simulink subsystem "Independent_Suspension_Double_Wishbone"  (R2024b)
settings: Solver=VariableStepAuto  StartTime=0.0  StopTime=10.0  RelTol=1e-3
model mask{ActiveDampEn=off, NumAxl=2, NumWhlsByAxl=[2 2], StrgEnByAxl=[1 0], AntiSwayEnByAxl=[0 0], WhlNumVec=[1  2  1  2], AxleNumVec=[1  1  2  2], SuspTypesByAxle=[1  1], SuspImage=suspdw.png, IdealSuspEn=on, IdealSuspAxles=[1  2], Kz=64370, F0z=9810, Cz=10000, Hmax=0.5, f_act_susp_cz=[10000 10000;10000 10000], f_act_susp_duty_bpt=[0 1], f_act_susp_zdot_bpt=[-1 1], Toe=0.0349, RollStrgSlp=-0.2269, ToeStrgSlp=0.01, Caster=0.0698, CasterHslp=-0.2269, CasterStrgSlp=0.01, Camber=0.0698, CamberHslp=-0.2269, CamberStrgSlp=0.01, StrgHgtSlp=0.1432, MappedSuspEn=off, MappedSuspAxles=[1  2], f_susp_axl_bp=[1 2], f_susp_dz_bp=[-0.15 -0.14 -0.13 -0.12 -0.11 -0.10 -0.09 -0.08 -0.07 -0.06 -0.05 -0.04 -0.03 -0.02 -0.01 0.00 0.01 0.02 0.03 0.04 0.05 0.06 0.07 0.08 0.09 0.10 0.11 0.12 0.13 0.14 0.15], f_susp_dzdot_bp=[-0.15 -0.14 -0.13 -0.12 -0.11 -0.10 -0.09 -0.08 -0.07 -0.06 -0.05 -0.04 -0.03 -0.02 -0.01 0.00 0.01 0.02 0.03 0.04 0.05 0.06 0.07 0.08 0.09 0.10 0.11 0.12 0.13 0.14 0.15], f_susp_fmz=zeros(31,31,61,2,4), f_susp_geom=zeros(31,61,2,3), f_susp_strgdelta_bp=[-30,-29,-28,-27,-26,-25,-24,-23,-22,-21,-20,-19,-18,-17,-16,-15,-14,-13,-12,-11,-10,-9,-8,-7,-6,-5,-4,-3,-2,-1,0,1,2,3,4,5,6,7,8,9,10,11,12,13,14,15,16,17,18,19,20,21,22,23,24,25,26,27,28,29,30], AntiSwayR=0.2, AntiSwayNtrlAng=0.5236, AntiSwayTrsK=5.7296e+03}
  mask prompts: ActiveDampEn "vdynblks:vehdynDoubleWishboneSuspension:blkDlg_ActiveDampEn"; NumAxl "vdynblks:vehdynDoubleWishboneSuspension:blkPrm_NumAxl"; NumWhlsByAxl "vdynblks:vehdynDoubleWishboneSuspension:blkPrm_NumWhlsByAxl"; StrgEnByAxl "vdynblks:vehdynDoubleWishboneSuspension:blkPrm_StrgEnByAxl"; AntiSwayEnByAxl "vdynblks:vehdynDoubleWishboneSuspension:blkPrm_AntiSwayEnByAxl"; WhlNumVec "vdynblks:vehdynDoubleWishboneSuspension:blkPrm_WhlNumVec"; AxleNumVec "vdynblks:vehdynDoubleWishboneSuspension:blkPrm_AxleNumVec"; SuspTypesByAxle "vdynblks:vehdynDoubleWishboneSuspension:blkPrm_SuspTypesByAxle"; SuspImage "vdynblks:vehdynDoubleWishboneSuspension:blkPrm_SuspImage"; IdealSuspEn "vdynblks:vehdynDoubleWishboneSuspension:blkPrm_IdealSuspEn"; IdealSuspAxles "vdynblks:vehdynDoubleWishboneSuspension:blkPrm_IdealSuspAxles"; Kz "vdynblks:vehdynDoubleWishboneSuspension:blkPrm_Kz"; F0z "vdynblks:vehdynDoubleWishboneSuspension:blkPrm_F0z"; Cz "vdynblks:vehdynDoubleWishboneSuspension:blkPrm_Cz"; Hmax "vdynblks:vehdynDoubleWishboneSuspension:blkPrm_Hmax"; f_act_susp_cz "vdynblks:vehdynDoubleWishboneSuspension:blkPrm_f_act_susp_cz"; f_act_susp_duty_bpt "vdynblks:vehdynDoubleWishboneSuspension:blkPrm_f_act_susp_duty_bpt"; f_act_susp_zdot_bpt "vdynblks:vehdynDoubleWishboneSuspension:blkPrm_f_act_susp_zdot_bpt"; Toe "vdynblks:vehdynDoubleWishboneSuspension:blkPrm_Toe"; RollStrgSlp "vdynblks:vehdynDoubleWishboneSuspension:blkPrm_RollStrgSlp"; ToeStrgSlp "vdynblks:vehdynDoubleWishboneSuspension:blkPrm_ToeStrgSlp"; Caster "vdynblks:vehdynDoubleWishboneSuspension:blkPrm_Caster"; CasterHslp "vdynblks:vehdynDoubleWishboneSuspension:blkPrm_CasterHslp"; CasterStrgSlp "vdynblks:vehdynDoubleWishboneSuspension:blkPrm_CasterStrgSlp"; Camber "vdynblks:vehdynDoubleWishboneSuspension:blkPrm_Camber"; CamberHslp "vdynblks:vehdynDoubleWishboneSuspension:blkPrm_CamberHslp"; CamberStrgSlp "vdynblks:vehdynDoubleWishboneSuspension:blkPrm_CamberStrgSlp"; StrgHgtSlp "vdynblks:vehdynDoubleWishboneSuspension:blkPrm_StrgHgtSlp"; MappedSuspEn "vdynblks:vehdynDoubleWishboneSuspension:blkPrm_MappedSuspEn"; MappedSuspAxles "vdynblks:vehdynDoubleWishboneSuspension:blkPrm_MappedSuspAxles"; f_susp_axl_bp "vdynblks:vehdynDoubleWishboneSuspension:blkPrm_f_susp_axl_bp"; f_susp_dz_bp "vdynblks:vehdynDoubleWishboneSuspension:blkPrm_f_susp_dz_bp"; f_susp_dzdot_bp "vdynblks:vehdynDoubleWishboneSuspension:blkPrm_f_susp_dzdot_bp"; f_susp_fmz "vdynblks:vehdynDoubleWishboneSuspension:blkPrm_f_susp_fmz"; f_susp_geom "vdynblks:vehdynDoubleWishboneSuspension:blkPrm_f_susp_geom"; f_susp_strgdelta_bp "vdynblks:vehdynDoubleWishboneSuspension:blkPrm_f_susp_strgdelta_bp"; AntiSwayR "vdynblks:vehdynDoubleWishboneSuspension:blkPrm_AntiSwayR"; AntiSwayNtrlAng "vdynblks:vehdynDoubleWishboneSuspension:blkPrm_AntiSwayNtrlAng"; AntiSwayTrsK "vdynblks:vehdynDoubleWishboneSuspension:blkPrm_AntiSwayTrsK"
undefined symbols (not defined in the file or in its folder): TrackCoords
libraries: vehdynlibsuspensioncommon x2
settings Model: Creator=blatak  LastModifiedBy=blatak

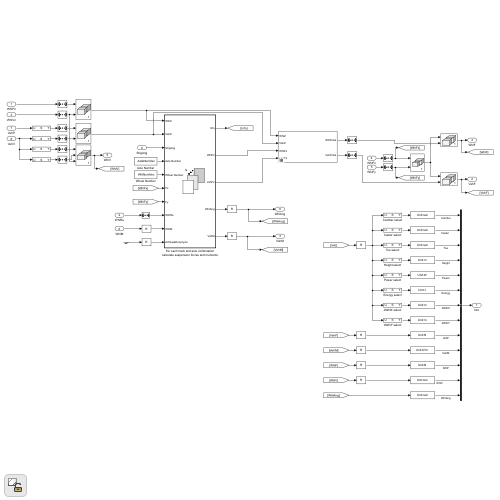
[thumbnail: Simulink's stored preview of the top-level diagram]
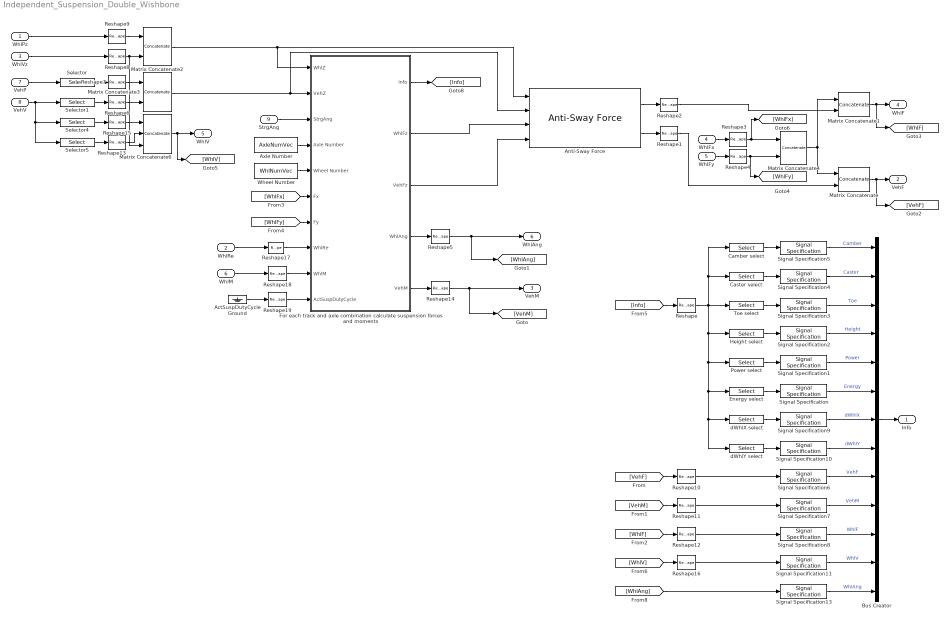
== system Independent_Suspension_Double_Wishbone ==
  WhlPz : Inport  Unit=m  PortDimensions=[1,length(WhlNumVec)]
  WhlRe : Inport  Port=2  Unit=m  PortDimensions=[1,length(WhlNumVec)]
  WhlVz : Inport  Port=3  Unit=m/s  PortDimensions=[1,length(WhlNumVec)]
  WhlFx : Inport  Port=4  Unit=N  PortDimensions=[1,length(WhlNumVec)]
  WhlFy : Inport  Port=5  Unit=N  PortDimensions=[1,length(WhlNumVec)]
  WhlM : Inport  Port=6  Unit=N*m  PortDimensions=[3,length(WhlNumVec)]
  VehP : Inport  Port=7  Unit=m  PortDimensions=[3,length(WhlNumVec)]
  VehV : Inport  Port=8  Unit=m/s  PortDimensions=[3,length(WhlNumVec)]
  StrgAng : Inport  Port=9  Unit=rad  PortDimensions=[1,sum(StrgEnByAxl.*NumWhlsByAxl)]
  ActSuspDutyCycle Ground : Ground
  Anti-Sway Force : vehdynlibsuspensioncommon/Anti-Sway Force  SystemSampleTime=-1  LabelModeActiveChoice=NoOp  VariantActivationTime=update diagram  AllowFlexibleInterface=on  Latency=0  AutoFrameSizeCalculation=off
      settings: LibrarySourceBlock=vehdynlibsuspension/Independent Suspension - Double Wishbone/Anti-Sway Force
  Axle Number : Constant  Value=AxleNumVec
  Bus Creator : BusCreator  Inputs=13
  Camber select : Selector  NumberOfDimensions=2  InputPortWidth=3  IndexOptions=Index vector (dialog),Select all  Indices=1,1  OutputSizes=1,1
  Caster select : Selector  NumberOfDimensions=2  InputPortWidth=3  IndexOptions=Index vector (dialog),Select all  Indices=2,1  OutputSizes=1,1
  Energy select : Selector  NumberOfDimensions=2  InputPortWidth=3  IndexOptions=Index vector (dialog),Select all  Indices=6,1  OutputSizes=1,1
  For each track and axle combination calculate suspension forces and moments : Subsystem  TreatAsAtomicUnit=on
  Height select : Selector  NumberOfDimensions=2  InputPortWidth=3  IndexOptions=Index vector (dialog),Select all  Indices=4,1  OutputSizes=1,1
  Matrix Concatenate{,1..4} (5 alike) : Concatenate  Mode=Multidimensional array
  Matrix Concatenate6 : Concatenate  NumInputs=3  Mode=Multidimensional array
  Power select : Selector  NumberOfDimensions=2  InputPortWidth=3  IndexOptions=Index vector (dialog),Select all  Indices=5,1  OutputSizes=1,1
  Reshape : Reshape  OutputDimensionality=Customize  OutputDimensions=[8,length(WhlNumVec)]
  Reshape{1..4,6..9,13,15,17} (11 alike) : Reshape  OutputDimensionality=Row vector (2-D)  OutputDimensions=[3,2*size(TrackCoords,1)]
  Reshape{5,10..12,14,16,18} (7 alike) : Reshape  OutputDimensionality=Customize  OutputDimensions=[3,length(WhlNumVec)]
  Reshape19 : Reshape  OutputDimensionality=Customize  OutputDimensions=[1,length(WhlNumVec)]
  Selector : Selector  NumberOfDimensions=2  InputPortWidth=3  IndexOptions=Index vector (dialog),Select all  Indices=3,1  OutputSizes=1,1
  Selector1 : Selector  NumberOfDimensions=2  InputPortWidth=3  IndexOptions=Index vector (dialog),Select all  Indices=3,1  OutputSizes=1,1
  Selector4 : Selector  NumberOfDimensions=2  InputPortWidth=3  IndexOptions=Index vector (dialog),Select all  Indices=1,1  OutputSizes=1,1
  Selector5 : Selector  NumberOfDimensions=2  InputPortWidth=3  IndexOptions=Index vector (dialog),Select all  Indices=2,1  OutputSizes=1,1
  Signal Specification : SignalSpecification  Unit=J
  Signal Specification1 : SignalSpecification  Unit=W
  Signal Specification10 : SignalSpecification  Unit=m
  Signal Specification11 : SignalSpecification  Unit=m/s
  Signal Specification{3..5,13} (4 alike) : SignalSpecification  Unit=rad
  Signal Specification2 : SignalSpecification  Unit=m
  Signal Specification6 : SignalSpecification  Unit=N
  Signal Specification7 : SignalSpecification  Unit=N*m
  Signal Specification8 : SignalSpecification  Unit=N
  Signal Specification9 : SignalSpecification  Unit=m
  Toe select : Selector  NumberOfDimensions=2  InputPortWidth=3  IndexOptions=Index vector (dialog),Select all  Indices=3,1  OutputSizes=1,1
  Wheel Number : Constant  Value=WhlNumVec
  dWhlX select : Selector  NumberOfDimensions=2  InputPortWidth=3  IndexOptions=Index vector (dialog),Select all  Indices=7,1  OutputSizes=1,1
  dWhlY select : Selector  NumberOfDimensions=2  InputPortWidth=3  IndexOptions=Index vector (dialog),Select all  Indices=8,1  OutputSizes=1,1
  Info : Outport  VectorParamsAs1DForOutWhenUnconnected=off
  VehF : Outport  Port=2  Unit=N  VectorParamsAs1DForOutWhenUnconnected=off
  VehM : Outport  Port=3  Unit=N*m  VectorParamsAs1DForOutWhenUnconnected=off
  WhlF : Outport  Port=4  Unit=N  VectorParamsAs1DForOutWhenUnconnected=off
  WhlV : Outport  Port=5  Unit=m/s  VectorParamsAs1DForOutWhenUnconnected=off
  WhlAng : Outport  Port=6  Unit=rad  VectorParamsAs1DForOutWhenUnconnected=off
  wires:
  Reshape3/1 -> Matrix Concatenate4/1, [WhlFx]
  [WhlFy] -> For each track and axle combination calculate suspension forces and moments/7(Fy)
  Reshape9/1 -> Matrix Concatenate2/1
  WhlM/1 -> Reshape18/1
  WhlPz/1 -> Reshape9/1
  For each track and axle combination calculate suspension forces and moments/3(VehFz) -> Anti-Sway Force/4
  [WhlFx] -> For each track and axle combination calculate suspension forces and moments/6(Fx)
  Matrix Concatenate3/1 -> Anti-Sway Force/2, For each track and axle combination calculate suspension forces and moments/2(VehZ)
  [WhlV] -> Reshape16/1
  Reshape14/1 -> [VehM], VehM/1
  Camber select/1 -> Signal Specification5/1
  Reshape2/1 -> Matrix Concatenate1/2
  Wheel Number/1 -> For each track and axle combination calculate suspension forces and moments/5(Wheel Number)
  VehV/1 -> Selector1/1, Selector4/1, Selector5/1
  Matrix Concatenate/1 -> VehF/1, [VehF]
  For each track and axle combination calculate suspension forces and moments/2(WhlFz) -> Anti-Sway Force/3
  Bus Creator/1 -> Info/1
  Reshape5/1 -> [WhlAng], WhlAng/1
  Matrix Concatenate4/1 -> Matrix Concatenate/1, Matrix Concatenate1/1
  [WhlAng] -> Signal Specification13/1
  Toe select/1 -> Signal Specification3/1
  Anti-Sway Force/1 -> Reshape2/1
  [VehM] -> Reshape11/1
  WhlFy/1 -> Reshape4/1
  Power select/1 -> Signal Specification1/1
  WhlFx/1 -> Reshape3/1
  Selector1/1 -> Reshape6/1
  Signal Specification/1 -> Bus Creator/6  "Energy"
  WhlVz/1 -> Reshape8/1
  [Info] -> Reshape/1
  Signal Specification7/1 -> Bus Creator/10  "VehM"
  VehP/1 -> Selector/1
  Height select/1 -> Signal Specification2/1
  Caster select/1 -> Signal Specification4/1
  Energy select/1 -> Signal Specification/1
  Reshape16/1 -> Signal Specification11/1
  Reshape1/1 -> Matrix Concatenate/2
  Reshape8/1 -> Matrix Concatenate6/3, Matrix Concatenate2/2
  Signal Specification8/1 -> Bus Creator/11  "WhlF"
  Reshape6/1 -> Matrix Concatenate3/2
  StrgAng/1 -> For each track and axle combination calculate suspension forces and moments/3(StrgAng)
  Matrix Concatenate6/1 -> WhlV/1, [WhlV]
  Reshape4/1 -> Matrix Concatenate4/2, [WhlFy]
  Selector/1 -> Reshape7/1
  Selector5/1 -> Reshape13/1
  For each track and axle combination calculate suspension forces and moments/1(Info) -> [Info]
  Signal Specification5/1 -> Bus Creator/1  "Camber"
  Axle Number/1 -> For each track and axle combination calculate suspension forces and moments/4(Axle Number)
  Signal Specification4/1 -> Bus Creator/2  "Caster"
  Reshape12/1 -> Signal Specification8/1
  Matrix Concatenate1/1 -> WhlF/1, [WhlF]
  Reshape10/1 -> Signal Specification6/1
  Reshape7/1 -> Matrix Concatenate3/1
  Reshape13/1 -> Matrix Concatenate6/2
  Signal Specification2/1 -> Bus Creator/4  "Height"
  Signal Specification3/1 -> Bus Creator/3  "Toe"
  [WhlF] -> Reshape12/1
  Signal Specification13/1 -> Bus Creator/13  "WhlAng"
  [VehF] -> Reshape10/1
  Signal Specification1/1 -> Bus Creator/5  "Power"
  For each track and axle combination calculate suspension forces and moments/5(VehM) -> Reshape14/1
  Signal Specification11/1 -> Bus Creator/12  "WhlV"
  WhlRe/1 -> Reshape17/1
  Selector4/1 -> Reshape15/1
  Signal Specification6/1 -> Bus Creator/9  "VehF"
  Reshape15/1 -> Matrix Concatenate6/1
  Anti-Sway Force/2 -> Reshape1/1
  Matrix Concatenate2/1 -> Anti-Sway Force/1, For each track and axle combination calculate suspension forces and moments/1(WhlZ)
  For each track and axle combination calculate suspension forces and moments/4(WhlAng) -> Reshape5/1
  Reshape11/1 -> Signal Specification7/1
  ActSuspDutyCycle Ground/1 -> Reshape19/1
  Reshape19/1 -> For each track and axle combination calculate suspension forces and moments/10(ActSuspDutyCycle)
  Reshape17/1 -> For each track and axle combination calculate suspension forces and moments/8(WhlRe)
  Reshape18/1 -> For each track and axle combination calculate suspension forces and moments/9(WhlM)
  Reshape/1 -> Toe select/1, Caster select/1, Camber select/1, Power select/1, Energy select/1, dWhlX select/1, dWhlY select/1, Height select/1
  Signal Specification10/1 -> Bus Creator/8  "dWhlY"
  dWhlX select/1 -> Signal Specification9/1
  Signal Specification9/1 -> Bus Creator/7  "dWhlX"
  dWhlY select/1 -> Signal Specification10/1

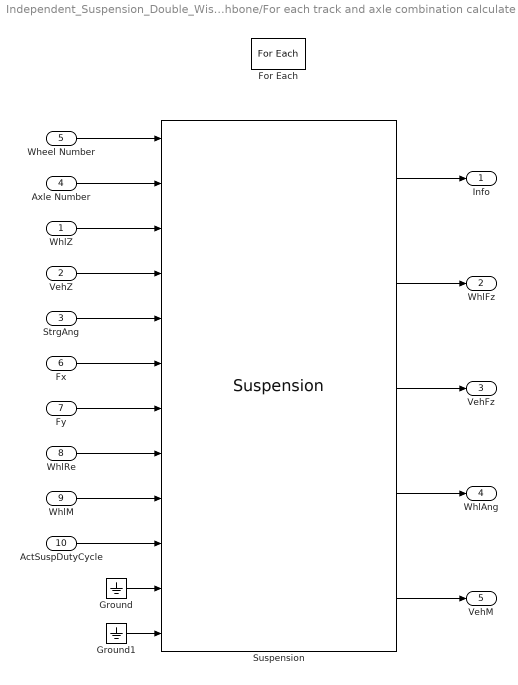
== system Independent_Suspension_Double_Wishbone/For each track and axle combination calculate suspension forces and moments ==
  WhlZ : Inport
  VehZ : Inport  Port=2
  StrgAng : Inport  Port=3
  Axle Number : Inport  Port=4  Partition=on  PartitionDimension=1  PartitionWidth=1  PartitionOffset=0
  Wheel Number : Inport  Port=5  Partition=on  PartitionDimension=1  PartitionWidth=1  PartitionOffset=0
  Fx : Inport  Port=6
  Fy : Inport  Port=7
  WhlRe : Inport  Port=8
  WhlM : Inport  Port=9
  ActSuspDutyCycle : Inport  Port=10  Unit=1  PortDimensions=[1,length(WhlNumVec)]
  For Each : ForEach  DisableCoverage=on
  Ground : Ground
  Ground1 : Ground
  Suspension : vehdynlibsuspensioncommon/Suspension  SystemSampleTime=-1  VariantControl=Ideal  VariantActivationTime=update diagram  AllowFlexibleInterface=on  Latency=0  AutoFrameSizeCalculation=off
      link override Suspension Angle Calculations: LabelModeActiveChoice=IdealSteeringEnabled
      link override Z axis suspension characteristic: LabelModeActiveChoice=IdealSuspension
      link override Z axis suspension characteristic/Ideal Suspension/Steering Height Slope: LabelModeActiveChoice=SteeringEnabled
  Info : Outport  ConcatenationDimension=1  VectorParamsAs1DForOutWhenUnconnected=off
  WhlFz : Outport  Port=2  ConcatenationDimension=1  VectorParamsAs1DForOutWhenUnconnected=off
  VehFz : Outport  Port=3  ConcatenationDimension=1  VectorParamsAs1DForOutWhenUnconnected=off
  WhlAng : Outport  Port=4  ConcatenationDimension=1  VectorParamsAs1DForOutWhenUnconnected=off
  VehM : Outport  Port=5  ConcatenationDimension=1  VectorParamsAs1DForOutWhenUnconnected=off
  wires:
  Ground1/1 -> Suspension/12
  Ground/1 -> Suspension/11
  ActSuspDutyCycle/1 -> Suspension/10
  Suspension/5 -> VehM/1
  WhlM/1 -> Suspension/9
  WhlRe/1 -> Suspension/8
  Fy/1 -> Suspension/7
  Fx/1 -> Suspension/6
  Suspension/4 -> WhlAng/1
  Suspension/3 -> VehFz/1
  Suspension/2 -> WhlFz/1
  StrgAng/1 -> Suspension/5
  VehZ/1 -> Suspension/4
  WhlZ/1 -> Suspension/3
  Wheel Number/1 -> Suspension/1
  Axle Number/1 -> Suspension/2
  Suspension/1 -> Info/1
